simulink library "UserBlocks"  (R2014a)
settings: Solver=ode45  SolverMode=SingleTasking  StartTime=0.0  StopTime=10.0  RelTol=1e-3
values from neighbouring files (symbols this model uses):
  a = param.a    [DSC_Control_Analysis.m]    (also in DSC_Control_Analysis_Exp.m; DSC_Speed_Control_Analysis.m; EmpiricalTireCurves.m = 1.35; FFW_Fx.m = sqrt(curvature/(2*clothoidLength)))
  b = 1.15    [EmpiricalTireCurves.m]
  Cfls = Cfl    [EC_params_nissan.m]
  Crls = Crl    [EC_params_nissan.m]
  d0 = CSTR.d0    [Ext_MPCPara.m]
  freq = Fs/2*linspace(0,1,NFFT/2)    [AACplottingcode.m]    (also in If_alpha_tp_observer.m; If_alpha_tp_observer_for_c_code.m; If_alpha_tp_observer_shoreline.m)
  Iz = param.Iz    [DSC_Control_Analysis.m]    (also in DSC_Control_Analysis_Exp.m; DSC_Speed_Control_Analysis.m; EmpiricalTireCurves.m = 1300)
  K = 10    [EC_params_nissan.m]
  Ks = -10    [EC_params_nissan.m]
  Ksl = -10    [EC_params_nissan.m]
  Kt = 40000    [EC_params_nissan.m]
  Ku = -40000    [EC_params_nissan.m]
  m = 1724    [EmpiricalTireCurves.m]
  mu_s = mu_p    (= 0.6)    [EC_params_nissan.m]    (also in EmpiricalTireCurves.m = 0.55)
  Ns = 10    [EC_params_nissan.m]
  num = num+MTnum(m)    [Build_MtMuMy.m]
  q = 1    [EC_params_nissan.m]
  Taoh = CSTR.Taoh    [Ext_MPCPara.m]
  Ts = 0.002    [DSC_Control_Analysis.m]    (also in DSC_Control_Analysis_Exp.m; DSC_Speed_Control_Analysis.m; EC_params_nissan.m; Ext_MPCPara.m = SSD.Ts)
undefined symbols (not defined in the file or in its folder): acceAmp, ack, alphaFrontSteeringLimit, alphaFrontTable, bit, c, Cfl, Crl, CSTR, dden, deltaPsiDotGain, deltDist, den, denafilt, dnum, elaDotGain, filtera, filterb, frontAlphaLookup, frontForceLookup, FuelStartCalTime, FyFtable, gpsins, h, h_roll, hal_filter_den, hal_filter_num, hwx, hwy5, initAcce, initSpeed, isDriverNoise, lkparams, mapDataFull, mapMatchingParams, maxFrontForce, maxNumSegs, mdPtrs, numafilt, param, rearAlphaLookup, rfl, rfr, rrl, rrr, sglu, SIMP, simuCond, slimFxl, slimFxu, sliml, slimMll, slimMlr, slimMul, slimMur, slimu, sr, SSD, Standard, steering_limit ... (+7)
libraries: simulink x28, slrtlib x18, UserBlocks x6, slrtsoftinglib x6, MickLibBlocks x1, DriftControllerLibrary x1
(part 3 of 6)

== system UserBlocks/Diagnostic System/Detection/Current Error ==
  Signal : Inport
  Abs : Abs  SaturateOnIntegerOverflow=on
  Constant : Constant  Value=thresh
  Relational Operator : RelationalOperator  OutDataTypeStr=float('double')
  Exceeds Threshold : Outport
  wires:
  Constant/1 -> Relational Operator/2
  Abs/1 -> Relational Operator/1
  Relational Operator/1 -> Exceeds Threshold/1
  Signal/1 -> Abs/1

== system UserBlocks/Diagnostic System/Detection/Gearbox Error ==
  Signal : Inport
  Abs : Abs  SaturateOnIntegerOverflow=on
  Constant : Constant  Value=thresh
  Relational Operator : RelationalOperator  OutDataTypeStr=float('double')
  Exceeds Threshold : Outport
  wires:
  Constant/1 -> Relational Operator/2
  Abs/1 -> Relational Operator/1
  Relational Operator/1 -> Exceeds Threshold/1
  Signal/1 -> Abs/1

== system UserBlocks/Diagnostic System/Detection/Motor Constant Error ==
  Signal : Inport
  Abs : Abs  SaturateOnIntegerOverflow=on
  Constant : Constant  Value=thresh
  Relational Operator : RelationalOperator  OutDataTypeStr=float('double')
  Exceeds Threshold : Outport
  wires:
  Constant/1 -> Relational Operator/2
  Abs/1 -> Relational Operator/1
  Relational Operator/1 -> Exceeds Threshold/1
  Signal/1 -> Abs/1

== system UserBlocks/Diagnostic System/Detection/Resistance Error ==
  Signal : Inport
  Abs : Abs  SaturateOnIntegerOverflow=on
  Constant : Constant  Value=thresh
  Relational Operator : RelationalOperator  OutDataTypeStr=float('double')
  Exceeds Threshold : Outport
  wires:
  Signal/1 -> Abs/1
  Relational Operator/1 -> Exceeds Threshold/1
  Abs/1 -> Relational Operator/1
  Constant/1 -> Relational Operator/2

== system UserBlocks/Diagnostic System/Detection/Steering Error ==
  Signal : Inport
  Abs : Abs  SaturateOnIntegerOverflow=on
  Constant : Constant  Value=thresh
  Relational Operator : RelationalOperator  OutDataTypeStr=float('double')
  Exceeds Threshold : Outport
  wires:
  Signal/1 -> Abs/1
  Relational Operator/1 -> Exceeds Threshold/1
  Abs/1 -> Relational Operator/1
  Constant/1 -> Relational Operator/2

== system UserBlocks/Diagnostic System/Detection/Yaw Rate Error A ==
  Signal : Inport
  Abs : Abs  SaturateOnIntegerOverflow=on
  Constant : Constant  Value=thresh
  Relational Operator : RelationalOperator  OutDataTypeStr=float('double')
  Exceeds Threshold : Outport
  wires:
  Signal/1 -> Abs/1
  Relational Operator/1 -> Exceeds Threshold/1
  Abs/1 -> Relational Operator/1
  Constant/1 -> Relational Operator/2

== system UserBlocks/Diagnostic System/Detection/Yaw Rate Error B ==
  Signal : Inport
  Abs : Abs  SaturateOnIntegerOverflow=on
  Constant : Constant  Value=thresh
  Relational Operator : RelationalOperator  OutDataTypeStr=float('double')
  Exceeds Threshold : Outport
  wires:
  Constant/1 -> Relational Operator/2
  Abs/1 -> Relational Operator/1
  Relational Operator/1 -> Exceeds Threshold/1
  Signal/1 -> Abs/1

== system UserBlocks/Diagnostic System/Detection/Yaw Rate Error C ==
  Signal : Inport
  Abs : Abs  SaturateOnIntegerOverflow=on
  Constant : Constant  Value=thresh
  Relational Operator : RelationalOperator  OutDataTypeStr=float('double')
  Exceeds Threshold : Outport
  wires:
  Signal/1 -> Abs/1
  Relational Operator/1 -> Exceeds Threshold/1
  Abs/1 -> Relational Operator/1
  Constant/1 -> Relational Operator/2

== system UserBlocks/Diagnostic System/Filtering/Another low-pass filter ==
  In1 : Inport
  Demux : Demux  Outputs=2
  Discrete Filter : DiscreteFilter  Numerator=num  Denominator=den  SampleTime=Ts
  Discrete Filter1 : DiscreteFilter  Numerator=num  Denominator=den  SampleTime=Ts
  Mux : Mux  Inputs=2
  Out1 : Outport
  wires:
  Demux/1 -> Discrete Filter/1
  Demux/2 -> Discrete Filter1/1
  Discrete Filter/1 -> Mux/1
  Discrete Filter1/1 -> Mux/2
  In1/1 -> Demux/1
  Mux/1 -> Out1/1

== system UserBlocks/Diagnostic System/Filtering/Low-pass filter ==
  In1 : Inport
  Demux : Demux  Outputs=2
  Discrete Filter : DiscreteFilter  Numerator=num  Denominator=den  SampleTime=Ts
  Discrete Filter1 : DiscreteFilter  Numerator=num  Denominator=den  SampleTime=Ts
  Mux : Mux  Inputs=2
  Out1 : Outport
  wires:
  Mux/1 -> Out1/1
  In1/1 -> Demux/1
  Discrete Filter1/1 -> Mux/2
  Discrete Filter/1 -> Mux/1
  Demux/2 -> Discrete Filter1/1
  Demux/1 -> Discrete Filter/1

== system UserBlocks/Diagnostic System/Residual Generation/Amplifier Model ==
  "Steering Motors " : Inport
  Current Commands : Inport  Port=2
  Bus Selector2 : BusSelector  OutputSignals=Currents
  Sum : Sum  Inputs=|-+  SaturateOnIntegerOverflow=on
  B : Outport
  wires:
  "Steering Motors "/1 -> Bus Selector2/1
  Sum/1 -> B/1
  Current Commands/1 -> Sum/1
  Bus Selector2/1 -> Sum/2  "<Currents>"

== system UserBlocks/Diagnostic System/Residual Generation/Controller Model ==
  "Steering Motors " : Inport
  Handwheel : Inport  Port=2
  Ackermann Correction : Subsystem
  Bus Selector2 : BusSelector  OutputSignals=Angles
  Software Steering Limit : Saturate  UpperLimit=steering_limit*pi/180  LowerLimit=-steering_limit*pi/180
  Steering Geometry & Gearbox Correction : Subsystem
      mask init:
      | p1_params
      | nissan_steer_lookup_data
  Steering Ratio : Gain  Gain=1/sr  SaturateOnIntegerOverflow=on  OutDataTypeStr=Inherit: Same as input  ParamDataTypeStr=Inherit: Same as input
  Sum : Sum  Inputs=|-+  SaturateOnIntegerOverflow=on
  filter : DiscreteFilter  Numerator=[wc*2*pi*Ts]  Denominator=[1 wc*2*pi*Ts-1]  SampleTime=Ts
  B : Outport
  wires:
  "Steering Motors "/1 -> Bus Selector2/1
  Bus Selector2/1 -> Sum/2  "<Angles>"
  Steering Ratio/1 -> Software Steering Limit/1
  Software Steering Limit/1 -> Ackermann Correction/1(Ackermann Angle)
  filter/1 -> Steering Ratio/1
  Handwheel/1 -> filter/1
  Sum/1 -> B/1
  Ackermann Correction/1(Steer Angles) -> Steering Geometry & Gearbox Correction/1(Steer Angles)
  Steering Geometry & Gearbox Correction/1(Shaft Angles) -> Sum/1

== system UserBlocks/Diagnostic System/Residual Generation/Gearbox Model ==
  "Steering Motors " : Inport
  Bus Selector2 : BusSelector  OutputSignals=Angles,Gearbox Angles
  Steering Ratio : Gain  Gain=[1/param.fl.gr ; 1/param.fr.gr]  SaturateOnIntegerOverflow=on  OutDataTypeStr=Inherit: Same as input  ParamDataTypeStr=Inherit: Same as input
  Sum : Sum  Inputs=+-|  SaturateOnIntegerOverflow=on
  A : Outport
  wires:
  Bus Selector2/1 -> Steering Ratio/1  "<Angles>"
  "Steering Motors "/1 -> Bus Selector2/1
  Sum/1 -> A/1
  Bus Selector2/2 -> Sum/2  "<Gearbox Angles>"
  Steering Ratio/1 -> Sum/1

== system UserBlocks/Diagnostic System/Residual Generation/Motor Parameter Estimators ==
  Steering Motors : Inport
  Current Commands : Inport  Port=2
  Bus Selector : BusSelector  OutputSignals=Voltages,Angles,Currents
  Demux : Demux  Outputs=2
  Demux1 : Demux  Outputs=2
  Demux2 : Demux  Outputs=2
  Derivative : Derivative
  Left Motor Estimator : S-Function  FunctionName=ckf  Parameters=V, [W(1) W(2) W(4)]  EnableBusSupport=off  mask{V=1000, W=[ 0.0001 0 ; 0 0.00005 ]}
      mask prompts: V "Measurement Noise:"; W "Process Noise:"
      mask Display:
      | port_label('output',1,'R');
      | port_label('output',2,'k');
      | port_label('output',3,'P');
      | port_label('input',1,'v');
      | port_label('input',2,'i');
      | port_label('input',3,'w');
  Mux : Mux  Inputs=2
  Mux1 : Mux  Inputs=2
  Nominal R : Constant  Value=[param.fl.Rm ; param.fr.Rm]
  Nominal k : Constant  Value=[param.fl.km ; param.fr.km]
  Right Motor Estimator : S-Function  FunctionName=rlsfilt  Parameters=lambda  EnableBusSupport=off  mask{lambda=.998}
      mask prompts: lambda "Forgetting Factor:"
      mask Display:
      | port_label('output',1,'R');
      | port_label('output',2,'k');
      | port_label('output',3,'P');
      | port_label('input',1,'v');
      | port_label('input',2,'i');
      | port_label('input',3,'w');
      | disp(sprintf('RLS Estimator\nlambda = %g',lambda));
  Sum : Sum  Inputs=|+-  SaturateOnIntegerOverflow=on
  Sum1 : Sum  Inputs=|+-  SaturateOnIntegerOverflow=on
  T1 : Terminator
  T2 : Terminator
  T3 : Terminator
  Resistances : Outport
  Motor Constants : Outport  Port=2
  wires:
  Bus Selector/1 -> Demux/1  "<Voltages>"
  Demux/1 -> Left Motor Estimator/1
  Demux/2 -> Right Motor Estimator/1
  Demux1/1 -> Left Motor Estimator/2
  Demux1/2 -> Right Motor Estimator/2
  Derivative/1 -> Demux2/1
  Bus Selector/2 -> Derivative/1  "<Angles>"
  Demux2/1 -> Left Motor Estimator/3
  Demux2/2 -> Right Motor Estimator/3
  Left Motor Estimator/1 -> Mux/1
  Left Motor Estimator/2 -> Mux1/1
  Right Motor Estimator/2 -> Mux1/2
  Mux/1 -> Sum/1
  Mux1/1 -> Sum1/1
  Nominal R/1 -> Sum/2
  Nominal k/1 -> Sum1/2
  Steering Motors/1 -> Bus Selector/1
  Sum/1 -> Resistances/1
  Sum1/1 -> Motor Constants/1
  Right Motor Estimator/3 -> T1/1
  Left Motor Estimator/3 -> T2/1
  Right Motor Estimator/1 -> Mux/2
  Bus Selector/3 -> Demux1/1  "<Currents>"
  Current Commands/1 -> T3/1

== system UserBlocks/Diagnostic System/Residual Generation/Select: Yaw Rate ==
  In1 : Inport
  Gain : Gain  Gain=K  Multiplication=Matrix(K*u)  SaturateOnIntegerOverflow=on  OutDataTypeStr=Inherit: Same as input  ParamDataTypeStr=Inherit: Same as input
  Out1 : Outport
  wires:
  Gain/1 -> Out1/1
  In1/1 -> Gain/1

== system UserBlocks/EnvEnv Connection/Compute delta Steer/100 Hz Trigger ==
  note: Eps is added before the floor to prevent numerical issues
  Clock : Clock
  Constant : Constant  Value=0.01
  Detect Change : simulink/Logic and Bit Operations/Detect Change  vinit=0  InputProcessing=Inherited  OutDataTypeStr=uint8
  Product : Product  Inputs=*/  RndMeth=Zero
  Rounding Function : Rounding
  Sum : Sum  Inputs=|++
  eps : Constant  Value=0.00001
  Out : Outport
  wires:
  eps/1 -> Sum/2
  Sum/1 -> Rounding Function/1
  Product/1 -> Sum/1
  Detect Change/1 -> Out/1
  Rounding Function/1 -> Detect Change/1
  Constant/1 -> Product/2
  Clock/1 -> Product/1

== system UserBlocks/EnvEnv Connection/Compute delta Steer/Check Comms ==
  note: Missed msg is defined as not receiving the
      | previous message before the next message is sent
  enableCL : Inport
  prevMsgNum : Inport  Port=2
  lastRecvMsgNum : Inport  Port=3
  Enable : EnablePort
  Compare To Zero1 : simulink/Logic and Bit Operations/Compare To Zero  relop===  OutDataTypeStr=uint8  ZeroCross=off
  Data Type Conversion1 : DataTypeConversion
  Data Type Conversion2 : DataTypeConversion
  Logical Operator1 : Logic  AllPortsSameDT=off  OutDataTypeStr=boolean
  Relational Operator : RelationalOperator  Operator=~=  OutDataTypeStr=boolean
  Sum1 : Sum  Inputs=|++
  Unit Delay2 : UnitDelay  SampleTime=-1
  commOkay : Outport
  numMissedMsg : Outport  Port=2
  wires:
  lastRecvMsgNum/1 -> Relational Operator/2
  enableCL/1 -> Logical Operator1/1
  Data Type Conversion2/1 -> commOkay/1
  prevMsgNum/1 -> Relational Operator/1
  Compare To Zero1/1 -> Data Type Conversion2/1
  Data Type Conversion1/1 -> Sum1/1
  Sum1/1 -> numMissedMsg/1, Unit Delay2/1, Compare To Zero1/1
  Unit Delay2/1 -> Sum1/2
  Logical Operator1/1 -> Data Type Conversion1/1
  Relational Operator/1 -> Logical Operator1/2

== system UserBlocks/EnvEnv Connection/Compute delta Steer/Cone Placer and Comms Status ==
  note: Read in cone
      | placer info and
      | msg counts to confirm
      | active comms
  Receive : slrtlib/UDP/Receive   ipAddress=171.64.164.232  ipPort=25012  width=4*8  vblLen=off  sampletime=-1
  Terminator : Terminator
  Unpack1 : slrtlib/UDP/Unpack   dimensions={4}  datatypes={'double'}  byteAlign=1
  Info : Outport
  wires:
  Receive/2 -> Terminator/1  "msgRecv"
  Unpack1/1 -> Info/1
  Receive/1 -> Unpack1/1

== system UserBlocks/EnvEnv Connection/Compute delta Steer/MPC UDP Receive ==
  Abs : Abs
  Bus Creator : BusCreator  Inputs=13
  Compare To Constant : simulink/Logic and Bit Operations/Compare To Constant  relop=>  const=0.1  OutDataTypeStr=uint8  ZeroCross=off
  Constant : Constant
  Demux : Demux  Outputs=12
  Product1 : Product  RndMeth=Zero
  Receive : slrtlib/UDP/Receive   ipAddress=171.64.164.232  ipPort=25011  width=12*8  vblLen=off  sampletime=-1
  Sum : Sum  Inputs=+-|
  Unpack1 : slrtlib/UDP/Unpack   dimensions={12}  datatypes={'double'}  byteAlign=1
  optResults : Outport
  wires:
  [deltaAdd_rad] -> Product1/2
  Demux/6 -> Bus Creator/6  "numRoutes"
  Demux/2 -> [deltaAdd_rad]  "deltaAdd_rad"
  [fail] -> Sum/1
  Demux/12 -> Bus Creator/13  "driverIntent_kN"
  Demux/11 -> Bus Creator/12  "u0_kN"
  Demux/10 -> Bus Creator/11  "corrN"
  Demux/9 -> Bus Creator/10  "corrTs"
  Demux/8 -> Bus Creator/9  "checkSum"
  Demux/7 -> Bus Creator/8  "optU_kN"
  Bus Creator/1 -> optResults/1
  Compare To Constant/1 -> Product1/1
  Abs/1 -> Compare To Constant/1
  Sum/1 -> Abs/1
  Constant/1 -> Sum/2
  Product1/1 -> Bus Creator/2  "delta_steerCmdAdd"
  Demux/5 -> Bus Creator/5  "optObjVal"
  Demux/4 -> Bus Creator/4  "numIter"
  Demux/3 -> [fail], Bus Creator/3  "fail"
  Demux/1 -> Bus Creator/1  "msgNumber"
  Unpack1/1 -> Demux/1
  Receive/2 -> Bus Creator/7  "msgRecv"
  Receive/1 -> Unpack1/1

== system UserBlocks/EnvEnv Connection/Compute delta Steer/MPC UDP Send ==
  States : Inport
  enableMPC : Inport  Port=2
  prev_steeringAngle : Inport  Port=3
  driverIntent_steeringAngle : Inport  Port=4
  prev_corrN : Inport  Port=5
  Enable : EnablePort
  Bus Creator : BusCreator  Inputs=7
  Bus Selector : BusSelector  OutputSignals=VyCG,Yaw Rate,Vx,Yaw Angle,Pos N,Pos E
  Data Type Conversion : DataTypeConversion
  Data Type Conversion3 : DataTypeConversion
  Logic : Subsystem
  Logical Operator : Logic  OutDataTypeStr=boolean
  Mux : Mux  Inputs=6
  Start MPC Calculation : Subsystem  TreatAsAtomicUnit=on
  Sum : Sum  Inputs=|++
  Unit Delay1 : UnitDelay  SampleTime=-1
  Unit Delay2 : UnitDelay  SampleTime=-1
  Unit Delay3 : UnitDelay  SampleTime=-1
  SentData : Outport
  enableCL : Outport  Port=2
  prevMsgNum : Outport  Port=3
  wires:
  Logic/1(prev_corrN_OUT) -> Bus Creator/3  "prev_corrN"
  prev_corrN/1 -> Logic/1(prev_corrN)
  Unit Delay2/1 -> Bus Creator/2  "xNLprev"
  Unit Delay3/1 -> prevMsgNum/1, Sum/2
  Sum/1 -> Bus Creator/7, Unit Delay3/1  "msgNumber"
  Data Type Conversion3/1 -> Logical Operator/2, Unit Delay1/1
  Mux/1 -> Unit Delay2/1, Bus Creator/1  "xNL"
  Bus Selector/3 -> Mux/3  "<Vx>"
  Data Type Conversion/1 -> enableCL/1
  Logical Operator/1 -> Data Type Conversion/1
  Unit Delay1/1 -> Logical Operator/1
  enableMPC/1 -> Bus Creator/6, Sum/1, Data Type Conversion3/1, Logic/2(enableCL)  "enableMPC"
  Start MPC Calculation/1(SentData_OUT) -> SentData/1
  Bus Creator/1 -> Start MPC Calculation/1(SentData_IN)
  driverIntent_steeringAngle/1 -> Bus Creator/5  "driverIntent_steeringAngle"
  prev_steeringAngle/1 -> Bus Creator/4  "prev_steeringAngle"
  Bus Selector/6 -> Mux/6  "<Pos E>"
  Bus Selector/5 -> Mux/5  "<Pos N>"
  Bus Selector/4 -> Mux/4  "<Yaw Angle>"
  Bus Selector/2 -> Mux/2  "<Yaw Rate>"
  Bus Selector/1 -> Mux/1  "<VyCG>"
  States/1 -> Bus Selector/1

== system UserBlocks/EnvEnv Connection/Compute delta Steer/Pass Through ==
  In1 : Inport
  Trigger : TriggerPort
  Out1 : Outport
  wires:
  In1/1 -> Out1/1

== system UserBlocks/Envelope control with Differential drive/envelope controller with DD/Control switch ==
  Beta_sw (VEC_sw) : Inport
  CONT ON flag : Inport  Port=2
  "Front tire slip angle limit switch 0 : OFF, 1: ON" : Constant  Value=0
  Logical Operator2 : Logic  AllPortsSameDT=off  OutDataTypeStr=boolean
  Logical Operator3 : Logic  AllPortsSameDT=off  OutDataTypeStr=boolean
  Logical Operator4 : Logic  AllPortsSameDT=off  OutDataTypeStr=boolean
  Manual Switch : ManualSwitch
  "Safe area 0 : small, 1: large" : Constant
  "Slip limit control switch 0: OFF , 1: ON" : Constant  Value=0
  Step : Step  SampleTime=0
  "Tire envelope control switch 0: TEC OFF , 1: TEC ON" : Constant
  "Vehicle envelope control switch 0: VEC OFF, 1:VEC ON" : Constant
  "drive switch 0 : OFF(no driving force), 1 : ON" : Constant
  tag scope: Beta_lim_sw=global, Boundary_sw=global, D_sw=global, TEC_sw=global, VEC_sw=global, cont_flag=global, df_sw=global, sliplimit_sw=global
  wires:
  Beta_sw (VEC_sw)/1 -> [Beta_lim_sw]
  "Safe area 0 : small, 1: large"/1 -> [Boundary_sw]
  "Slip limit control switch 0: OFF , 1: ON"/1 -> Manual Switch/1
  Step/1 -> Manual Switch/2
  Manual Switch/1 -> [sliplimit_sw]
  "drive switch 0 : OFF(no driving force), 1 : ON"/1 -> [D_sw]
  Logical Operator3/1 -> [VEC_sw]
  Logical Operator2/1 -> [TEC_sw]
  Logical Operator4/1 -> [df_sw]
  "Tire envelope control switch 0: TEC OFF , 1: TEC ON"/1 -> Logical Operator2/2
  "Vehicle envelope control switch 0: VEC OFF, 1:VEC ON"/1 -> Logical Operator3/2
  "Front tire slip angle limit switch 0 : OFF, 1: ON"/1 -> Logical Operator4/2
  CONT ON flag/1 -> Logical Operator2/1, [cont_flag], Logical Operator4/1, Logical Operator3/1

== system UserBlocks/Envelope control with Differential drive/envelope controller with DD/Estimator switch ==
  "Beta estimation switch 0: from estimator, 1:from GPS" : Constant
  "Vx switch 0: from wheel speed, 1:from GPS" : Constant
  "lateral weight shift switch 0: OFF, 1:ON" : Constant
  "longitudinal weight shift swich 0: OFF, 1:ON" : Constant
  "muFz estimation switch 0: from estimator, 1:from GPS " : Constant
  tag scope: Vx_sw=global, ax_sw=global, ay_sw=global, beta_est_sw=global, muFz_est_sw=global
  wires:
  "Vx switch 0: from wheel speed, 1:from GPS"/1 -> [Vx_sw]
  "Beta estimation switch 0: from estimator, 1:from GPS"/1 -> [beta_est_sw]
  "muFz estimation switch 0: from estimator, 1:from GPS "/1 -> [muFz_est_sw]
  "longitudinal weight shift swich 0: OFF, 1:ON"/1 -> [ax_sw]
  "lateral weight shift switch 0: OFF, 1:ON"/1 -> [ay_sw]

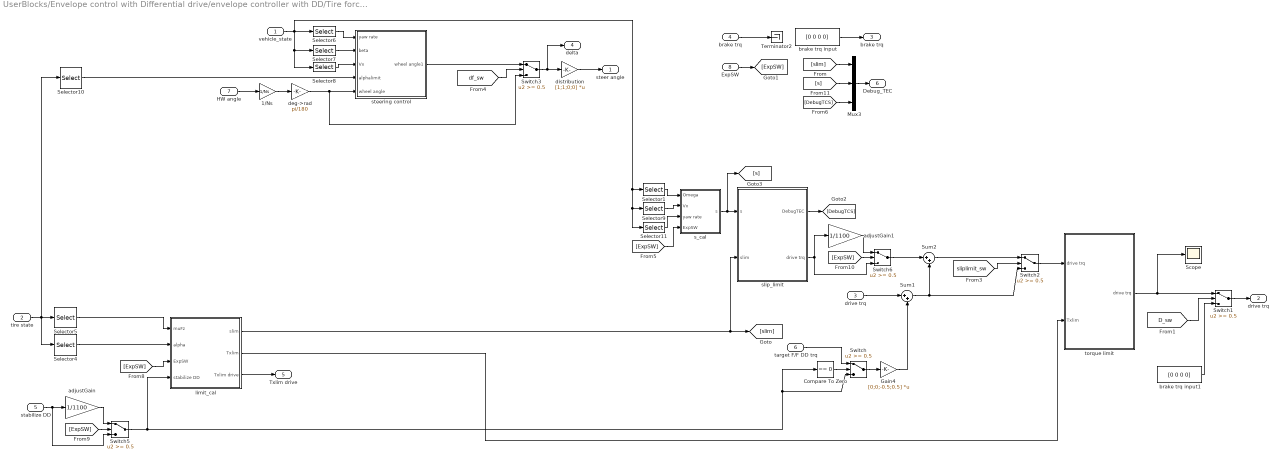
== system UserBlocks/Envelope control with Differential drive/envelope controller with DD/Tire force control ==
  vehicle_state : Inport
  tire state : Inport  Port=2
  "drive trq " : Inport  Port=3
  "brake trq " : Inport  Port=4
  stabilize DD : Inport  Port=5
  target F/F DD trq : Inport  Port=6
  HW angle : Inport  Port=7
  ExpSW : Inport  Port=8
  1/Ns : Gain  Gain=1/Ns
  Compare To Zero : simulink/Logic and Bit Operations/Compare To Zero  relop===  OutDataTypeStr=uint8  ZeroCross=off
  Gain4 : Gain  Gain=[0;0;-0.5;0.5]  Multiplication=Matrix(K*u)
  Mux3 : Mux  Inputs=3
  Scope : Scope
      settings: YMin=-200  YMax=225  SaveName=ScopeData8
  Selector1 : Selector  InputPortWidth=12  Indices=[1:4]
  Selector10 : Selector  InputPortWidth=9  Indices=[7:8]
  Selector11 : Selector  InputPortWidth=12  Indices=7
  Selector4 : Selector  InputPortWidth=9  Indices=[1:2]
  Selector5 : Selector  InputPortWidth=9  Indices=[3:6]
  Selector6 : Selector  InputPortWidth=12  Indices=7
  Selector7 : Selector  InputPortWidth=12  Indices=12
  Selector8 : Selector  InputPortWidth=12  Indices=5
  Selector9 : Selector  InputPortWidth=12  Indices=5
  Sum1 : Sum  Inputs=|++
  Sum2 : Sum  Inputs=|++
  Switch{,1..3,5..6} (6 alike) : Switch  Threshold=0.5
  Terminator2 : Terminator
  adjustGain : Gain  Gain=1/1100
  adjustGain1 : Gain  Gain=1/1100
  brake trq input : Constant  Value=[0 0 0 0]
  brake trq input1 : Constant  Value=[0 0 0 0]
  deg->rad : Gain  Gain=pi/180
  distribution : Gain  Gain=[1;1;0;0]  Multiplication=Matrix(K*u)
  limit_cal : Subsystem
  "s_cal " : Subsystem
  slip_limit : Subsystem
  steering control : Subsystem
  torque limit : Subsystem
  steer angle : Outport
  drive trq : Outport  Port=2
  brake trq : Outport  Port=3
  delta : Outport  Port=4
  Txlim drive : Outport  Port=5
  Debug_TEC : Outport  Port=6
  wires:
  target F/F DD trq/1 -> Switch/1
  Gain4/1 -> Sum1/2
  Compare To Zero/1 -> Switch/2
  "drive trq "/1 -> Sum1/1
  Switch5/1 -> Switch/3, Compare To Zero/1, limit_cal/4(stabilize DD)
  limit_cal/1(slim) -> [slim], slip_limit/2(slim)
  Switch2/1 -> torque limit/1("drive trq ")
  Sum1/1 -> Switch2/3, Sum2/2
  Sum2/1 -> Switch2/1
  Switch6/1 -> Sum2/1
  Switch/1 -> Gain4/1
  limit_cal/3(Txlim drive) -> Txlim drive/1
  [sliplimit_sw] -> Switch2/2
  [D_sw] -> Switch1/2
  brake trq input1/1 -> Switch1/3
  Switch1/1 -> drive trq/1
  "s_cal "/1(s) -> [s], slip_limit/1(s)
  Selector1/1 -> "s_cal "/1(Omega)
  "brake trq "/1 -> Terminator2/1
  brake trq input/1 -> brake trq/1
  tire state/1 -> Selector5/1, Selector4/1, Selector10/1
  limit_cal/2(Txlim) -> torque limit/2(Txlim)
  [df_sw] -> Switch3/2
  Switch3/1 -> distribution/1, delta/1
  steering control/1(wheel angle1) -> Switch3/1
  HW angle/1 -> 1/Ns/1
  distribution/1 -> steer angle/1
  1/Ns/1 -> deg->rad/1
  deg->rad/1 -> steering control/5(wheel angle), Switch3/3
  Selector8/1 -> steering control/3(Vx)
  Selector4/1 -> limit_cal/2(alpha)
  Selector5/1 -> limit_cal/1(muFz)
  vehicle_state/1 -> Selector6/1, Selector1/1, Selector9/1, Selector11/1, Selector7/1, Selector8/1
  Selector6/1 -> steering control/1(yaw rate)
  Selector7/1 -> steering control/2(beta)
  torque limit/1(drive trq) -> Switch1/1, Scope/1
  Selector9/1 -> "s_cal "/2(Vx)
  Selector10/1 -> steering control/4(alphalimit)
  slip_limit/1(DebugTEC) -> [DebugTCS]
  [slim] -> Mux3/1
  Mux3/1 -> Debug_TEC/1
  Selector11/1 -> "s_cal "/3(yaw rate)
  [ExpSW] -> "s_cal "/4(ExpSW)
  ExpSW/1 -> [ExpSW]
  [ExpSW] -> limit_cal/3(ExpSW)
  [ExpSW] -> Switch5/2
  stabilize DD/1 -> Switch5/3, adjustGain/1
  adjustGain/1 -> Switch5/1
  [ExpSW] -> Switch6/2
  adjustGain1/1 -> Switch6/1
  slip_limit/2(drive trq) -> adjustGain1/1, Switch6/3
  [DebugTCS] -> Mux3/3
  [s] -> Mux3/2

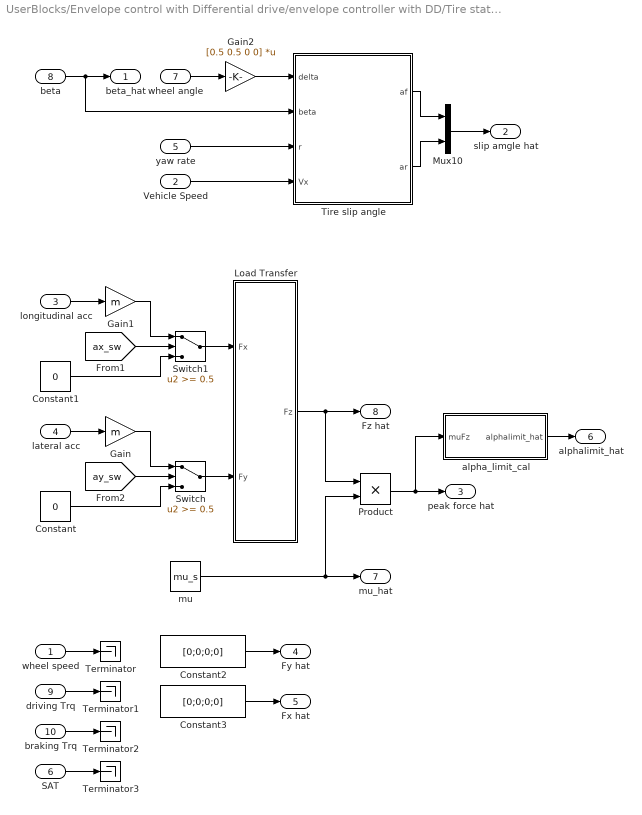
== system UserBlocks/Envelope control with Differential drive/envelope controller with DD/Tire state estimation ==
  wheel speed : Inport
  Vehicle Speed : Inport  Port=2
  longitudinal acc : Inport  Port=3
  lateral acc : Inport  Port=4
  yaw rate : Inport  Port=5
  SAT : Inport  Port=6
  wheel angle : Inport  Port=7
  beta : Inport  Port=8
  driving Trq : Inport  Port=9
  braking Trq : Inport  Port=10
  Constant : Constant  Value=0
  Constant1 : Constant  Value=0
  Constant2 : Constant  Value=[0;0;0;0]
  Constant3 : Constant  Value=[0;0;0;0]
  Gain : Gain  Gain=m
  Gain1 : Gain  Gain=m
  Gain2 : Gain  Gain=[0.5 0.5 0 0]  Multiplication=Matrix(K*u)
  Load Transfer : Subsystem
  Mux10 : Mux  Inputs=2
  Product : Product  RndMeth=Zero
  Switch : Switch  Threshold=0.5
  Switch1 : Switch  Threshold=0.5
  Terminator{,1..3} (4 alike) : Terminator
  Tire slip angle : Subsystem
  alpha_limit_cal : Subsystem
  mu : Constant  Value=mu_s
  beta_hat : Outport
  slip amgle hat : Outport  Port=2
  peak force hat : Outport  Port=3
  Fy hat : Outport  Port=4
  Fx hat : Outport  Port=5
  alphalimit_hat : Outport  Port=6
  mu_hat : Outport  Port=7
  Fz hat : Outport  Port=8
  wires:
  lateral acc/1 -> Gain/1
  Load Transfer/1(Fz) -> Fz hat/1, Product/1
  alpha_limit_cal/1(alphalimit_hat) -> alphalimit_hat/1
  Switch/1 -> Load Transfer/2(Fy)
  [ay_sw] -> Switch/2
  Constant/1 -> Switch/3
  Gain/1 -> Switch/1
  longitudinal acc/1 -> Gain1/1
  [ax_sw] -> Switch1/2
  Constant1/1 -> Switch1/3
  Gain1/1 -> Switch1/1
  Switch1/1 -> Load Transfer/1(Fx)
  mu/1 -> mu_hat/1, Product/2
  Product/1 -> peak force hat/1, alpha_limit_cal/1(muFz)
  beta/1 -> beta_hat/1, Tire slip angle/2(beta)
  wheel angle/1 -> Gain2/1
  Gain2/1 -> Tire slip angle/1(delta)
  yaw rate/1 -> Tire slip angle/3(r)
  Vehicle Speed/1 -> Tire slip angle/4(Vx)
  Tire slip angle/1(af) -> Mux10/1
  Tire slip angle/2(ar) -> Mux10/2
  Mux10/1 -> slip amgle hat/1
  wheel speed/1 -> Terminator/1
  driving Trq/1 -> Terminator1/1
  braking Trq/1 -> Terminator2/1
  SAT/1 -> Terminator3/1
  Constant2/1 -> Fy hat/1
  Constant3/1 -> Fx hat/1

== system UserBlocks/Envelope control with Differential drive/envelope controller with DD/VSP_cal ==
  wheel speed : Inport
  Vehicle Speed : Inport  Port=2
  Gain1 : Gain  Gain=[rfl rfr 0 0]/2  Multiplication=Matrix(K*u)
  Switch1 : Switch  Threshold=0.5
  Zero-Order Hold1 : ZeroOrderHold  SampleTime=0.002
  prevent zero : Subsystem
  VSP : Outport
  wires:
  [Vx_sw] -> Switch1/2
  Gain1/1 -> Switch1/3
  Switch1/1 -> prevent zero/1(In1)
  Zero-Order Hold1/1 -> Switch1/1
  Vehicle Speed/1 -> Zero-Order Hold1/1
  wheel speed/1 -> Gain1/1
  prevent zero/1(Out1) -> VSP/1

== system UserBlocks/Envelope control with Differential drive/envelope controller with DD/brake_dynamics ==
  In1 : Inport
  Demux : Demux
  Discrete Transfer Fcn{,1..3} (4 alike) : DiscreteTransferFcn  Numerator=0.3297  Denominator=[1 -0.6703]  SampleTime=0.002
  Mux : Mux
  Out1 : Outport
  wires:
  In1/1 -> Demux/1
  Mux/1 -> Out1/1
  Demux/1 -> Discrete Transfer Fcn/1
  Demux/2 -> Discrete Transfer Fcn1/1
  Demux/3 -> Discrete Transfer Fcn2/1
  Demux/4 -> Discrete Transfer Fcn3/1
  Discrete Transfer Fcn/1 -> Mux/1
  Discrete Transfer Fcn1/1 -> Mux/2
  Discrete Transfer Fcn2/1 -> Mux/3
  Discrete Transfer Fcn3/1 -> Mux/4

== system UserBlocks/Envelope control with Differential drive/envelope controller with DD/control_on ==
  note: [Control on condition]
      | - Switch ON
      | - Brake OFF
      | - Vx > 2m/s
      | - GPS works
  Fault switch : Inport
  brake_sw : Inport  Port=2
  Vx : Inport  Port=3
  Bus Selector1 : BusSelector  OutputSignals=Velocity Solution Status,Attitude Status
  Constant : Constant  Value=2
  Constant1 : Constant  Value=3
  Constant2 : Constant  Value=4
  Data Type Conversion1 : DataTypeConversion  OutDataTypeStr=double  RndMeth=Nearest  SaturateOnIntegerOverflow=on
  Data Type Conversion2 : DataTypeConversion  OutDataTypeStr=double  RndMeth=Nearest  SaturateOnIntegerOverflow=on
  Data Type Conversion3 : DataTypeConversion  RndMeth=Nearest  SaturateOnIntegerOverflow=on
  Logical Operator : Logic  Operator=NOT  AllPortsSameDT=off  OutDataTypeStr=boolean
  Logical Operator{1..4} (4 alike) : Logic  AllPortsSameDT=off  OutDataTypeStr=boolean
  Relational Operator : RelationalOperator  Operator=>  OutDataTypeStr=boolean
  Relational Operator1 : RelationalOperator  Operator===  OutDataTypeStr=boolean
  Relational Operator2 : RelationalOperator  Operator===  OutDataTypeStr=boolean
  Rounding Function : Rounding  Operator=round
  Rounding Function1 : Rounding  Operator=round
  ON FLAG : Outport
  tag scope: ECDDbrake=global, ECDDspeed=global, GPS_condition=global
  wires:
  brake_sw/1 -> Data Type Conversion3/1
  Fault switch/1 -> Logical Operator1/1
  Logical Operator/1 -> Logical Operator1/2
  Vx/1 -> Relational Operator/1
  Constant/1 -> Relational Operator/2
  Logical Operator1/1 -> Logical Operator2/1
  Relational Operator/1 -> Logical Operator2/2, [ECDDspeed]
  Bus Selector1/1 -> Data Type Conversion2/1  "<Velocity Solution Status>"
  Bus Selector1/2 -> Data Type Conversion1/1  "<Attitude Status>"
  [global_GPS] -> Bus Selector1/1
  Data Type Conversion2/1 -> Rounding Function/1
  Data Type Conversion1/1 -> Rounding Function1/1
  Rounding Function/1 -> Relational Operator1/2
  Constant1/1 -> Relational Operator1/1
  Rounding Function1/1 -> Relational Operator2/1
  Constant2/1 -> Relational Operator2/2
  Relational Operator1/1 -> Logical Operator3/1
  Relational Operator2/1 -> Logical Operator3/2
  Logical Operator2/1 -> Logical Operator4/1
  Logical Operator3/1 -> [GPS_condition], Logical Operator4/2
  Logical Operator4/1 -> ON FLAG/1
  Data Type Conversion3/1 -> Logical Operator/1, [ECDDbrake]

== system UserBlocks/Envelope control with Differential drive/envelope controller with DD/drive_dynamics ==
  In1 : Inport
  Demux : Demux
  Discrete Transfer Fcn{,1..3} (4 alike) : DiscreteTransferFcn  Numerator=0.3297  Denominator=[1 -0.6703]  SampleTime=0.002
  Mux : Mux
  Out1 : Outport
  wires:
  Discrete Transfer Fcn3/1 -> Mux/4
  Discrete Transfer Fcn2/1 -> Mux/3
  Discrete Transfer Fcn1/1 -> Mux/2
  Discrete Transfer Fcn/1 -> Mux/1
  Demux/4 -> Discrete Transfer Fcn3/1
  Demux/3 -> Discrete Transfer Fcn2/1
  Demux/2 -> Discrete Transfer Fcn1/1
  Demux/1 -> Discrete Transfer Fcn/1
  Mux/1 -> Out1/1
  In1/1 -> Demux/1

== system UserBlocks/Envelope control with Differential drive/envelope controller with DD/reaction force control ==
  reaction 1 : Inport
  reaction 2 : Inport  Port=2
  Constant : Constant  Value=0
  Constant1 : Constant  Value=0
  Constant2 : Constant  Value=0
  Terminator : Terminator
  Terminator1 : Terminator
  steer force : Outport
  ACC pedal force : Outport  Port=2
  Brake pedal force1 : Outport  Port=3
  wires:
  Constant/1 -> steer force/1
  Constant1/1 -> ACC pedal force/1
  Constant2/1 -> Brake pedal force1/1
  reaction 1/1 -> Terminator/1
  reaction 2/1 -> Terminator1/1

== system UserBlocks/Envelope control with Differential drive/envelope controller with DD/target making ==
  vehicle state : Inport
  APO : Inport  Port=2
  brake pedal : Inport  Port=3
  HW angle : Inport  Port=4
  ExpSW : Inport  Port=5
  Txlim drive : Inport  Port=6
  Constant1 : Constant  Value=0
  Constant2 : Constant  Value=0
  Constant3 : Constant  Value=0
  Diff_gain : Constant  Value=2
  Discrete Transfer Fcn : DiscreteTransferFcn  Numerator=dnum  Denominator=dden  SampleTime=0.002
  Gain1 : Gain  Gain=m
  Gain2 : Gain
  Gain3 : Gain  Gain=9.8
  Gain4 : Gain  Gain=[0;0;0.5*rrl;0.5*rrr]  Multiplication=Matrix(K*u)
  Gain5 : Gain
  Gain7 : Gain  Gain=[0;0;1;1]  Multiplication=Matrix(K*u)
  Lookup Table : Lookup  InputValues=[0;1;2;3]  Table=[0;0;1;1]
  Manual Switch : ManualSwitch  CurrentSetting=0
  Manual Switch1 : ManualSwitch  CurrentSetting=0
  Manual Switch2 : ManualSwitch
  Manual Switch3 : ManualSwitch
  Product : Product  RndMeth=Zero
  Product1 : Product  RndMeth=Zero
  Selector8 : Selector  InputPortWidth=12  Indices=5
  Switch : Switch  Threshold=0.5
  Switch5 : Switch  Threshold=0.5
  Terminator3 : Terminator
  adjustGain : Gain  Gain=1/1100
  driving_dynamics : Subsystem
      mask init:
      | fomg=1.5;
  torque limit : Subsystem
  target yaw rate : Outport
  target lateral acc : Outport  Port=2
  target F/F DD trq : Outport  Port=3
  target driving torque : Outport  Port=4
  wires:
  Manual Switch1/1 -> Manual Switch2/1
  Manual Switch3/1 -> Manual Switch1/2
  driving_dynamics/1(Out1) -> Manual Switch3/2
  Product1/1 -> driving_dynamics/1(In1), Manual Switch3/1
  Switch5/1 -> target F/F DD trq/1
  Product/1 -> Switch5/3, adjustGain/1
  adjustGain/1 -> Switch5/1
  Diff_gain/1 -> Product1/2
  Discrete Transfer Fcn/1 -> Product1/1
  Constant3/1 -> Manual Switch2/2
  Manual Switch2/1 -> Product/1
  Gain5/1 -> Manual Switch1/1
  Lookup Table/1 -> Product/2
  Selector8/1 -> Lookup Table/1
  vehicle state/1 -> Selector8/1
  Gain2/1 -> Discrete Transfer Fcn/1, Gain5/1
  HW angle/1 -> Gain2/1
  Constant2/1 -> target yaw rate/1
  Manual Switch/1 -> target driving torque/1
  torque limit/1(drive trq) -> Manual Switch/2
  Txlim drive/1 -> torque limit/2(Txlim drive)
  Switch/1 -> Manual Switch/1, torque limit/1("drive trq ")
  Gain7/1 -> Switch/1
  APO/1 -> Gain7/1, Gain1/1
  Gain4/1 -> Switch/3
  ExpSW/1 -> Switch5/2, Switch/2
  brake pedal/1 -> Terminator3/1
  Constant1/1 -> target lateral acc/1
  Gain1/1 -> Gain3/1
  Gain3/1 -> Gain4/1

== system UserBlocks/Envelope control with Differential drive/envelope controller with DD/vehicle motion control ==
  vehicle state : Inport
  tire state : Inport  Port=2
  motion target : Inport  Port=3
  ExpSW : Inport  Port=4
  delta : Inport  Port=5
  Slip : Inport  Port=6
  Constant{1..4} (4 alike) : Constant  Value=0
  EC : Subsystem
  GPS status : slrtlib/Displays and Logging/Scope   scopeno=4  scopetype=Target  autostart=on  viewmode=Graphical sliding  formatstr='%15.6f'  grid=on  ylimits=[-1,1]  nosamples=round(1/Ts)  noprepostsamples=0  interleave=1  triggermode=FreeRun  triggersignal=1  trigsignalfromport=off  triggerlevel=0.0  triggerslope=Either  triggerscope=1  triggersample=0  filename=data.dat  mode=Lazy  writesize=512  autorestart=off  dynamicfilemode=off  maxwritefilesize=512*1024^2
  GPS status1 : slrtlib/Displays and Logging/Scope   scopeno=5  scopetype=Target  autostart=on  viewmode=Graphical sliding  formatstr='%15.6f'  grid=on  ylimits=[-1,1]  nosamples=round(1/Ts)  noprepostsamples=0  interleave=1  triggermode=FreeRun  triggersignal=1  trigsignalfromport=off  triggerlevel=0.0  triggerslope=Either  triggerscope=1  triggersample=0  filename=data.dat  mode=Lazy  writesize=512  autorestart=off  dynamicfilemode=off  maxwritefilesize=512*1024^2
  Gain4 : Gain  Gain=[0;0;-0.5;0.5]  Multiplication=Matrix(K*u)
  Mux1 : Mux  Inputs=3
  Mux2 : Mux  Inputs=2
  Selector : Selector  InputPortWidth=7  Indices=[4:7]
  Selector1 : Selector  InputPortWidth=12  Indices=12
  Selector2 : Selector  InputPortWidth=12  Indices=7
  Selector3 : Selector  InputPortWidth=9  Indices=[7:8]
  Selector4 : Selector  InputPortWidth=12  Indices=5
  Selector5 : Selector  InputPortWidth=7  Indices=3
  Selector6 : Selector  InputPortWidth=9  Indices=[3:6]
  Selector7 : Selector  InputPortWidth=11  Indices=[8 9]
  Selector8 : Selector  InputPortWidth=11  Indices=[6 7]
  Selector9 : Selector  InputPortWidth=9  Indices=9
  Sum : Sum  Inputs=|++
  Switch3 : Switch  Threshold=0.5
  derive trq : Outport
  brake trq : Outport  Port=2
  stabilize DD : Outport  Port=3
  target F/F DD trq : Outport  Port=4
  reaction 1 : Outport  Port=5
  reaction 2 : Outport  Port=6
  Debug_VEC : Outport  Port=7
  wires:
  Sum/1 -> EC/10(drive_trq)
  Gain4/1 -> Sum/1
  Selector5/1 -> Gain4/1, target F/F DD trq/1
  Selector/1 -> Sum/2, derive trq/1
  Selector9/1 -> EC/5(mu_hat)
  Switch3/1 -> stabilize DD/1
  Slip/1 -> EC/9(Slip)
  ExpSW/1 -> EC/8(ExpSW)
  Selector6/1 -> EC/4(peak_force_hat)
  Selector8/1 -> Mux2/2
  Mux2/1 -> GPS status1/1
  Constant2/1 -> brake trq/1
  Constant3/1 -> reaction 1/1
  Constant4/1 -> reaction 2/1
  motion target/1 -> Selector5/1, Selector/1
  Selector2/1 -> Mux2/1, EC/1(yaw rate)
  vehicle state/1 -> Selector4/1, Selector2/1, Selector1/1
  Selector1/1 -> EC/2(beta), Mux1/1
  Selector3/1 -> Mux1/2, EC/3(alpha_limit)
  tire state/1 -> Selector9/1, Selector6/1, Selector3/1
  delta/1 -> EC/7(wheel angle)
  [VEC_sw] -> Switch3/2
  EC/2(target DD) -> Switch3/1
  Constant1/1 -> Switch3/3
  Selector4/1 -> EC/6(Vx)
  EC/1(DebugVEC) -> Selector8/1, Debug_VEC/1, Selector7/1
  Selector7/1 -> Mux1/3
  Mux1/1 -> GPS status/1

== system UserBlocks/LQACC/PIDACC/Car-Following System ==
  PVacce : Inport
  PVvel : Inport  Port=2
  vehSpd : Inport  Port=3
  vehAcce : Inport  Port=4
  Car-Follow Sys : Subsystem
  Mux : Mux  Inputs=3
  SysOut : Outport
  PV_acce : Outport  Port=2
  actDist : Outport  Port=3
  VehSpd : Outport  Port=4
  DesDist : Outport  Port=5
  wires:
  Mux/1 -> SysOut/1
  PVvel/1 -> Car-Follow Sys/1(preSpd)
  vehSpd/1 -> VehSpd/1, Car-Follow Sys/2(vehSpd)
  vehAcce/1 -> Car-Follow Sys/3(vehAcce)
  PVacce/1 -> PV_acce/1
  Car-Follow Sys/4(dist) -> actDist/1
  Car-Follow Sys/3(vehACCE) -> Mux/3
  Car-Follow Sys/2(relVel) -> Mux/2
  Car-Follow Sys/1(distErr) -> Mux/1
  Car-Follow Sys/5(DesDist) -> DesDist/1

== system UserBlocks/LQACC/PIDACC/MPC MTCACC ==
  SysOut : Inport
  PreAcce : Inport  Port=2
  actDist : Inport  Port=3
  vehSpd : Inport  Port=4
  MTC ACC control : Subsystem
  T : Terminator
  epsilon : Outport
  desAcce : Outport  Port=2
  wires:
  actDist/1 -> T/1
  PreAcce/1 -> MTC ACC control/1(PreAcce)
  SysOut/1 -> MTC ACC control/2(sysOuts)
  vehSpd/1 -> MTC ACC control/3(VehSpd)
  MTC ACC control/2(epsilon) -> epsilon/1
  MTC ACC control/1(desAcce) -> desAcce/1

== system UserBlocks/LQACC/PIDACC/PreVehicle ==
  Pattern : Inport
  Add : Sum  Inputs=+-
  Add1 : Sum  Inputs=+--+
  Add2 : Sum  Inputs=+-+-
  City Road StartTime=20s : Subsystem
  Const Vp : Constant  Value=Vpinit1
  Const Vp1 : Constant  Value=5
  Const Vp2 : Constant  Value=0.25
  Const Vp3 : Constant  Value=4
  Const Vp5 : Constant  Value=4
  Diff1 : Subsystem
  Express Way StartTime=20s : Subsystem
  Integrator1 : Integrator  InitialConditionSource=external
  Pulse Generator : DiscretePulseGenerator  PulseType=Time based  Amplitude=.5  Period=10  PulseWidth=50
  Ramp : simulink/Sources/Ramp  slope=.2  start=10  X0=0
  Ramp1 : simulink/Sources/Ramp  slope=.2  start=20  X0=0
  Ramp3 : simulink/Sources/Ramp  slope=.2  start=30  X0=0
  Ramp4 : simulink/Sources/Ramp  slope=.2  start=40  X0=0
  Sine Wave1 : Sin  Amplitude=.4  Frequency=.314  SampleTime=0
  Step : Step  Time=15  After=.2  SampleTime=0
  Step1 : Step  Time=25  After=.2  SampleTime=0
  Step2 : Step  Time=45  After=.2  SampleTime=0
  Step3 : Step  Time=55  After=.2  SampleTime=0
  Switch : MultiPortSwitch  Inputs=7  SaturateOnIntegerOverflow=on
  Switch1 : MultiPortSwitch  Inputs=7  SaturateOnIntegerOverflow=on
  initSlope : Subsystem
  initSlope3 : Subsystem
  sineAcce : Subsystem
  PreAcce : Outport
  PreSpeed : Outport  Port=2
  wires:
  Ramp4/1 -> Add2/4
  Ramp3/1 -> Add2/3
  Ramp1/1 -> Add2/2
  Ramp/1 -> Add2/1
  Step3/1 -> Add1/4
  Step2/1 -> Add1/3
  Step1/1 -> Add1/2
  Step/1 -> Add1/1
  Const Vp5/1 -> Switch1/5
  Const Vp2/1 -> Add/2
  Pulse Generator/1 -> Add/1
  Add/1 -> Switch/4
  Const Vp1/1 -> Switch1/4
  Integrator1/1 -> PreSpeed/1
  Switch1/1 -> Integrator1/2
  Sine Wave1/1 -> Switch/3
  Const Vp3/1 -> Switch1/3
  City Road StartTime=20s/2(Vlead) -> Switch1/7
  City Road StartTime=20s/1(Alead) -> Switch/7
  initSlope3/1(Xout) -> Switch1/6
  initSlope/1(Xout) -> Switch1/2, Diff1/1(x)
  Express Way StartTime=20s/1(Alead) -> Switch/8
  Express Way StartTime=20s/2(Vlead) -> Switch1/8
  Add2/1 -> Switch/6
  Add1/1 -> Switch/5
  Diff1/1(dx) -> Switch/2
  sineAcce/1(speed) -> initSlope3/1(Xin)
  Const Vp/1 -> initSlope/1(Xin)
  Switch/1 -> Integrator1/1, PreAcce/1
  Pattern/1 -> Switch/1, Switch1/1

== system UserBlocks/LQACC/PIDACC/Subsystem ==
  ax : Inport
  Constant : Constant  Value=0  SampleTime=Ts
  Gear Ratio : Gain  Gain=1/5.5  SampleTime=Ts
  Saturation : Saturate  UpperLimit=2.8  LowerLimit=0
  Sum : Sum  Inputs=|+-
  Torque2volt : Lookup  InputValues=[-90,0,210]  Table=[0,1.9,2.8]  LookUpMeth=Interpolation-Use End Values  SampleTime=Ts
  convert to force : Gain  Gain=m  SampleTime=Ts
  motor efficiency : Gain  Gain=1/.91  SampleTime=Ts
  "two motors " : Gain  Gain=1/2  SampleTime=Ts
  wheel radius : Gain  Gain=.32  SampleTime=Ts
  Volt(V)1 : Outport
  wires:
  convert to force/1 -> wheel radius/1  "force required"
  wheel radius/1 -> Gear Ratio/1  "torque required @ wheelS"
  Gear Ratio/1 -> motor efficiency/1
  motor efficiency/1 -> "two motors "/1  "torque required  @ motorS"
  Torque2volt/1 -> Sum/1
  ax/1 -> convert to force/1
  "two motors "/1 -> Torque2volt/1  "torque required  @ each motor"
  Sum/1 -> Saturation/1
  Saturation/1 -> Volt(V)1/1
  Constant/1 -> Sum/2  "remove offset as this offset will be add later in the switching logic block"

== system UserBlocks/MPCACC/PIDACC/Car-Following System ==
  PVacce : Inport
  PVvel : Inport  Port=2
  vehSpd : Inport  Port=3
  vehAcce : Inport  Port=4
  Car-Follow Sys : Subsystem
  Mux : Mux  Inputs=3
  SysOut : Outport
  PV_acce : Outport  Port=2
  actDist : Outport  Port=3
  VehSpd : Outport  Port=4
  DesDist : Outport  Port=5
  wires:
  Car-Follow Sys/5(DesDist) -> DesDist/1
  Car-Follow Sys/1(distErr) -> Mux/1
  Car-Follow Sys/2(relVel) -> Mux/2
  Car-Follow Sys/3(vehACCE) -> Mux/3
  Car-Follow Sys/4(dist) -> actDist/1
  PVacce/1 -> PV_acce/1
  vehAcce/1 -> Car-Follow Sys/3(vehAcce)
  vehSpd/1 -> Car-Follow Sys/2(vehSpd), VehSpd/1
  PVvel/1 -> Car-Follow Sys/1(preSpd)
  Mux/1 -> SysOut/1

== system UserBlocks/MPCACC/PIDACC/MPC MTCACC ==
  SysOut : Inport
  Prevel : Inport  Port=2
  actDist : Inport  Port=3
  vehSpd : Inport  Port=4
  mdPtrs : Inport  Port=5
  MTC ACC control : Subsystem
  T : Terminator
  epsilon : Outport
  desAcce : Outport  Port=2
  wires:
  actDist/1 -> T/1
  Prevel/1 -> MTC ACC control/3(Prevel)
  SysOut/1 -> MTC ACC control/2(sysOuts)
  vehSpd/1 -> MTC ACC control/4(VehVel)
  MTC ACC control/1(Ctrl) -> desAcce/1
  MTC ACC control/2(epsilon) -> epsilon/1
  mdPtrs/1 -> MTC ACC control/1(mdPtrs)

== system UserBlocks/MPCACC/PIDACC/Subsystem ==
  ax : Inport
  Constant : Constant  Value=0  SampleTime=Ts
  Gear Ratio : Gain  Gain=1/5.5  SampleTime=Ts
  Saturation : Saturate  UpperLimit=2.8  LowerLimit=0
  Sum : Sum  Inputs=|+-
  Torque2volt : Lookup  InputValues=[-90,0,210]  Table=[0,1.75,2.8]  LookUpMeth=Interpolation-Use End Values  SampleTime=Ts
  convert to force : Gain  Gain=m  SampleTime=Ts
  motor efficiency : Gain  Gain=1/.91  SampleTime=Ts
  "two motors " : Gain  Gain=1/2  SampleTime=Ts
  wheel radius : Gain  Gain=.32  SampleTime=Ts
  Volt(V)1 : Outport
  wires:
  Constant/1 -> Sum/2  "remove offset as this offset will be add later in the switching logic block"
  Saturation/1 -> Volt(V)1/1
  Sum/1 -> Saturation/1
  "two motors "/1 -> Torque2volt/1  "torque required  @ each motor"
  ax/1 -> convert to force/1
  Torque2volt/1 -> Sum/1
  motor efficiency/1 -> "two motors "/1  "torque required  @ motorS"
  Gear Ratio/1 -> motor efficiency/1
  wheel radius/1 -> Gear Ratio/1  "torque required @ wheelS"
  convert to force/1 -> wheel radius/1  "force required"

== system UserBlocks/Offline Estimation/Data Extractor/Motor Current Fixup Due to Voltage Limitation ==
  Motor Angles : Inport
  Current Commands : Inport  Port=2
  1/Rm L : Gain  Gain=1/param.fl.Rm
  1/Rm R : Gain  Gain=1/param.fr.Rm
  Demux : Demux  Outputs=2
  Demux1 : Demux  Outputs=2
  Gain4 : Gain  Gain=-1
  Gain7 : Gain  Gain=-1
  Left Omega : simulink/Discrete/Discrete Derivative  gainval=1.0  ICPrevScaledInput=0.0  InputProcessing=Inherited  OutMin=[]  OutMax=[]  OutDataType=sfix(16)  OutScaling=2^-10  DoSatur=off
  Max Voltage L : Constant  Value=param.fl.Vmax
  Max Voltage R : Constant  Value=param.fr.Vmax
  Mux1 : Mux  Inputs=2
  Right Omega : simulink/Discrete/Discrete Derivative  gainval=1.0  ICPrevScaledInput=0.0  InputProcessing=Inherited  OutMin=[]  OutMax=[]  OutDataType=sfix(16)  OutScaling=2^-10  DoSatur=off
  Rm L : Gain  Gain=param.fl.Rm
  Rm R : Gain  Gain=param.fr.Rm
  Sum : Sum  Inputs=+|+
  Sum1 : Sum  Inputs=+|+
  Sum2 : Sum  Inputs=|+-
  Sum3 : Sum  Inputs=|+-
  Voltage Saturation L : simulink/Discontinuities/Saturation Dynamic  OutMin=[]  OutMax=[]  OutDataTypeStr=Inherit: Same as second input  OutDataType=sfix(16)  OutScaling=2^-10  DoSatur=off
  Voltage Saturation R : simulink/Discontinuities/Saturation Dynamic  OutMin=[]  OutMax=[]  OutDataTypeStr=Inherit: Same as second input  OutDataType=sfix(16)  OutScaling=2^-10  DoSatur=off
  km L : Gain  Gain=param.fl.km
  km R : Gain  Gain=param.fr.km
  Motor Currents : Outport
  wires:
  Current Commands/1 -> Demux/1
  Demux/1 -> Rm L/1
  Demux/2 -> Rm R/1
  Left Omega/1 -> km L/1
  Right Omega/1 -> km R/1
  Rm L/1 -> Sum1/1
  km L/1 -> Sum1/2, Sum2/2
  Rm R/1 -> Sum/1
  km R/1 -> Sum/2, Sum3/2
  Sum/1 -> Voltage Saturation R/2
  Sum1/1 -> Voltage Saturation L/2
  Voltage Saturation L/1 -> Sum2/1
  Voltage Saturation R/1 -> Sum3/1
  Sum2/1 -> 1/Rm L/1
  Sum3/1 -> 1/Rm R/1
  1/Rm R/1 -> Mux1/2
  1/Rm L/1 -> Mux1/1
  Mux1/1 -> Motor Currents/1
  Max Voltage L/1 -> Gain4/1, Voltage Saturation L/1
  Max Voltage R/1 -> Gain7/1, Voltage Saturation R/1
  Gain7/1 -> Voltage Saturation R/3
  Gain4/1 -> Voltage Saturation L/3
  Demux1/1 -> Left Omega/1
  Demux1/2 -> Right Omega/1
  Motor Angles/1 -> Demux1/1

== system UserBlocks/Offline Estimation/Data Extractor/Select: Left Motor Angle ==
  In1 : Inport
  Gain : Gain  Gain=K  Multiplication=Matrix(K*u)  SaturateOnIntegerOverflow=on  OutDataTypeStr=Inherit: Same as input  ParamDataTypeStr=Inherit: Same as input
  Out1 : Outport
  wires:
  Gain/1 -> Out1/1
  In1/1 -> Gain/1

== system UserBlocks/Offline Estimation/Data Extractor/Select: Right Motor Angle ==
  In1 : Inport
  Gain : Gain  Gain=K  Multiplication=Matrix(K*u)  SaturateOnIntegerOverflow=on  OutDataTypeStr=Inherit: Same as input  ParamDataTypeStr=Inherit: Same as input
  Out1 : Outport
  wires:
  Gain/1 -> Out1/1
  In1/1 -> Gain/1

== system UserBlocks/Offline Estimation/Data Extractor/Select: Yaw Rate ==
  In1 : Inport
  Gain : Gain  Gain=K  Multiplication=Matrix(K*u)  SaturateOnIntegerOverflow=on  OutDataTypeStr=Inherit: Same as input  ParamDataTypeStr=Inherit: Same as input
  Out1 : Outport
  wires:
  Gain/1 -> Out1/1
  In1/1 -> Gain/1

== system UserBlocks/Offline Estimation/Data Extractor/Steering Geometry & Gearbox Correction ==
  Motor Angles : Inport
  Demux : Demux  Outputs=2
  Left Steer Angle Look-up : Lookup  InputValues=sglu.fl.ma  SaturateOnIntegerOverflow=on
  Mux4 : Mux  Inputs=2
  Right Steer Angle Look-up : Lookup  InputValues=sglu.fr.ma  SaturateOnIntegerOverflow=on
  Steering Ratio : Gain  Gain=1/param.fr.gr  SaturateOnIntegerOverflow=on  OutDataTypeStr=Inherit: Same as input  ParamDataTypeStr=Inherit: Same as input
  Steering Ratio1 : Gain  Gain=1/param.fl.gr  SaturateOnIntegerOverflow=on  OutDataTypeStr=Inherit: Same as input  ParamDataTypeStr=Inherit: Same as input
  Steer Angles : Outport
  wires:
  Left Steer Angle Look-up/1 -> Mux4/1
  Right Steer Angle Look-up/1 -> Mux4/2
  Mux4/1 -> Steer Angles/1
  Motor Angles/1 -> Demux/1
  Demux/1 -> Steering Ratio1/1
  Demux/2 -> Steering Ratio/1
  Steering Ratio/1 -> Right Steer Angle Look-up/1
  Steering Ratio1/1 -> Left Steer Angle Look-up/1

== system UserBlocks/Sliding Surface Control Subsystem/Sliding Surface Controller function/get_d_control ==
  B : Inport
  Vx : Inport  Port=2
  r : Inport  Port=3
  alphaFcontrol : Inport  Port=4
  Gain : Gain  Gain=a
  Product1 : Product  RndMeth=Zero
  Sum : Sum  Inputs=|++
  Sum1 : Sum  Inputs=|+-
  Trigonometric Function : Trigonometry  Operator=atan2
  d_control : Outport
  wires:
  Product1/1 -> Sum/1
  Gain/1 -> Sum/2
  Sum/1 -> Trigonometric Function/1
  B/1 -> Product1/1
  r/1 -> Gain/1
  Vx/1 -> Product1/2, Trigonometric Function/2
  Trigonometric Function/1 -> Sum1/1
  alphaFcontrol/1 -> Sum1/2
  Sum1/1 -> d_control/1

== system UserBlocks/Sliding Surface Control Subsystem v1/Sliding Surface Controller function/Kcontrol ==
  Vx : Inport
  Constant : Constant  Value=10
  Gain : Gain  Gain=0
  Saturation : Saturate  UpperLimit=20  LowerLimit=5
  Sum : Sum  Inputs=|+-
  Kcontrol : Outport
  wires:
  Sum/1 -> Saturation/1
  Vx/1 -> Gain/1
  Constant/1 -> Sum/1
  Gain/1 -> Sum/2
  Saturation/1 -> Kcontrol/1

== system UserBlocks/Sliding Surface Control Subsystem v1/Sliding Surface Controller function/getFyf_control ==
  r : Inport
  Vx : Inport  Port=2
  Fyr : Inport  Port=3
  rnomdot : Inport  Port=4
  Bnomdot : Inport  Port=5
  Surface_S : Inport  Port=6
  Kcontrol : Inport  Port=7
  Add : Sum  Inputs=+++++
  Constant1 : Constant
  Constant2 : Constant  Value=a/Iz
  Divide : Product  Inputs=*/
  Divide1 : Product  Inputs=/*
  Gain : Gain  Gain=-q
  Gain1 : Gain  Gain=-q
  Gain2 : Gain  Gain=-1
  Gain3 : Gain  Gain=q/m
  Gain4 : Gain  Gain=b/Iz
  Product : Product  RndMeth=Zero
  Product1 : Product  RndMeth=Zero
  Saturation : Saturate  UpperLimit=maxFrontForce  LowerLimit=-maxFrontForce
  Sum : Sum  Inputs=|++
  Sum1 : Sum  Inputs=|-+
  Fyfcontrol : Outport
  wires:
  Saturation/1 -> Fyfcontrol/1
  Divide1/1 -> Saturation/1
  Divide/1 -> Gain3/1
  Constant1/1 -> Divide/1
  Vx/1 -> Divide/2
  r/1 -> Gain1/1
  Add/1 -> Divide1/2
  Sum1/1 -> Divide1/1
  Constant2/1 -> Sum1/2
  Sum/1 -> Add/2
  Gain4/1 -> Sum/2
  Product/1 -> Sum/1
  Fyr/1 -> Gain4/1, Product/2
  Gain3/1 -> Sum1/1, Product/1
  Gain1/1 -> Add/1
  rnomdot/1 -> Add/3
  Gain/1 -> Add/4
  Product1/1 -> Add/5
  Surface_S/1 -> Product1/1
  Bnomdot/1 -> Gain/1
  Kcontrol/1 -> Gain2/1
  Gain2/1 -> Product1/2
